simulink model "pulse_code_modulation"  (R2020a)
settings: Solver=VariableStepAuto  StartTime=0.0  StopTime=10.0  RelTol=1e-3
libraries: commutil2 x2, dspquant2 x2, dsparch4 x1, dspsigops x1
settings Model: Creator=91735  LastModifiedBy=91735

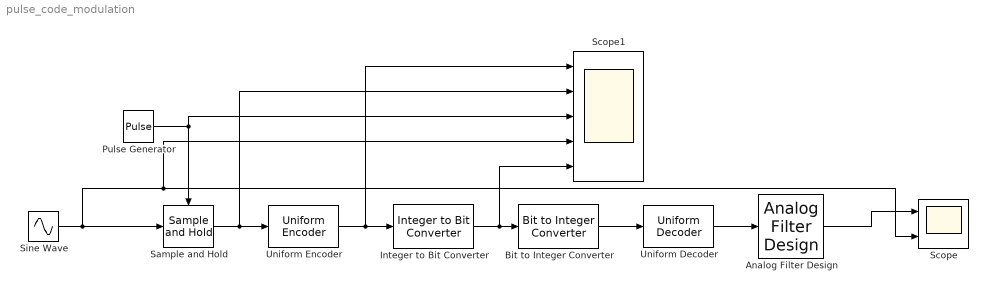
== system pulse_code_modulation ==
  Analog Filter Design : dsparch4/Analog Filter Design  method=Butterworth  filttype=Lowpass  N=8  Wlo=2*pi*2  Whi=80  Rp=2  Rs=40
  Bit to Integer Converter : commutil2/Bit to Integer Converter  nbits=3  bitOrder=MSB first  signedOutputValues=Signed  outDtype=Inherit via internal rule  outDtypeSigned=Inherit via internal rule
  Integer to Bit Converter : commutil2/Integer to Bit Converter  nbits=3  signedInputValues=Signed  bitOrder=MSB first  outDtype=Inherit via internal rule
  Pulse Generator : DiscretePulseGenerator  PulseType=Time based  Amplitude=5  Period=1/20  PulseWidth=50
  Sample and Hold : dspsigops/Sample and Hold  trig=Rising edge  initCond=0  latchinput=off
  Scope : Scope  NumInputPorts=2
  Scope1 : Scope  NumInputPorts=5
  Sine Wave : Sin  Amplitude=5  Frequency=2*pi*2  SampleTime=0
  Uniform Decoder : dspquant2/Uniform Decoder  peak=5  bits=3  overflowMode=Saturate  otype=Double
      settings: SourceProductBaseCode=DS
  Uniform Encoder : dspquant2/Uniform Encoder  peak=5  bits=3  otype=Signed integer
  wires:
  Uniform Encoder/1 -> Scope1/1, Integer to Bit Converter/1
  Sample and Hold/1 -> Scope1/2, Uniform Encoder/1
  Integer to Bit Converter/1 -> Scope1/5, Bit to Integer Converter/1
  Uniform Decoder/1 -> Analog Filter Design/1
  Bit to Integer Converter/1 -> Uniform Decoder/1
  Analog Filter Design/1 -> Scope/1
  Pulse Generator/1 -> Sample and Hold/Trigger, Scope1/3
  Sine Wave/1 -> Scope1/4, Scope/2, Sample and Hold/1
